simulink model "Output_ROS"  (R2022b)
settings: Solver=FixedStepAuto  StartTime=0.0  StopTime=128  FixedStep=0.02  RelTol=1e-3
undefined symbols (not defined in the file): b, unicycle, X, Y
libraries: robotlib x3, simulink_extras x1
settings Model: Creator=mustacchim  LastModifiedBy=mustacchim
settings OptimizationCC: EnhancedBackFolding=on  PassReuseOutputArgsAs=Individual arguments  ZeroExternalMemoryAtStartup=off  ZeroInternalMemoryAtStartup=off  MaxStackSize=64  OptimizeBlockOrder=speed  DifferentSizesBufferReuse=on  OptimizationCustomize=off  EfficientTunableParamExpr=on
settings DebuggingCC: ParameterTunabilityLossMsg=error
settings HardwareCC: ProdBitPerPointer=32  ProdBitPerSizeT=32  ProdBitPerPtrDiffT=32  ProdLargestAtomicFloat=None  ProdIntDivRoundTo=Undefined  ProdEndianess=Unspecified  ProdWordSize=32  ProdHWDeviceType=Generic->Unspecified (assume 32-bit Generic)
settings SFSimCC: MATLABDynamicMemAlloc=off
settings RTWCC: Description=Embedded Coder  SystemTargetFile=ert.tlc  HardwareBoard=Robot Operating System (ROS)  TLCOptions="-aInlineSetEventsForThisBaseRateFcn=TLC_FALSE -aSuppressMultiTaskScheduler=TLC_FALSE  -aRateBasedStepFcn=0"  TemplateMakefile=ert_default_tmf  Toolchain=Catkin  TargetLang=C++
settings CodeAppCC: ForceParamTrailComments=on  IgnoreCustomStorageClasses=off  OperatorAnnotations=on  SimulinkDataObjDesc=on  SFDataObjDesc=on  InsertBlockDesc=on

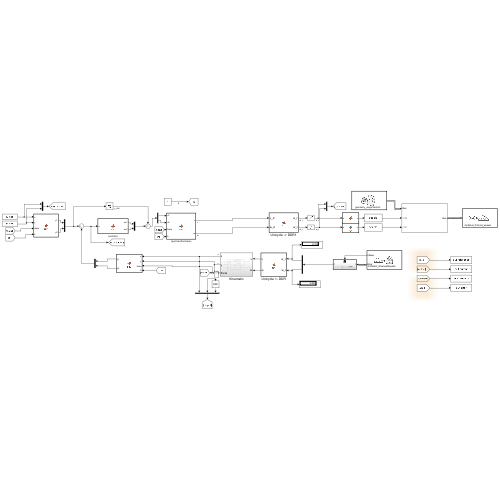
[thumbnail: Simulink's stored preview of the top-level diagram]
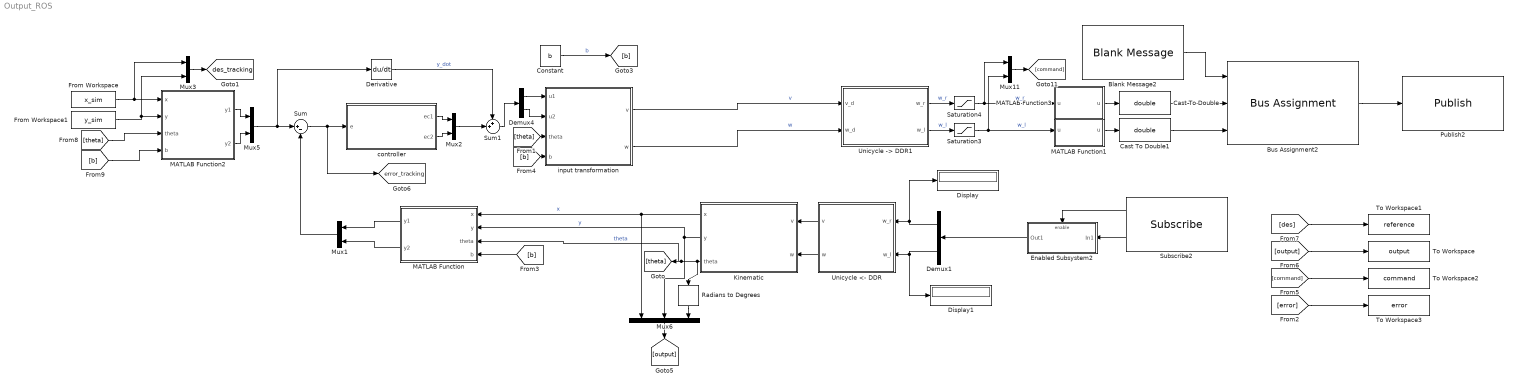
== system Output_ROS ==
  Blank Message2 : robotlib/Blank Message  messageClass=Message  entityType=geometry_msgs/Vector3  messageType=geometry_msgs/Vector3  SampleTime=0.02  legacyBusStruct=off
      settings: LibrarySourceBlock=roslib/ROS/Blank Message
  Bus Assignment2 : BusAssignment  AssignedSignals=X,Y
  Cast To Double : DataTypeConversion  OutDataTypeStr=double  SaturateOnIntegerOverflow=off  RndMeth=Floor
  Cast To Double1 : DataTypeConversion  OutDataTypeStr=double  SaturateOnIntegerOverflow=off  RndMeth=Floor
  Constant : Constant  Value=b
  Demux1 : Demux  Outputs=2
  Demux4 : Demux  Outputs=2
  Derivative : Derivative
  Display : Display
  Display1 : Display
  Enabled Subsystem2 : Subsystem  TreatAsAtomicUnit=on
  From Workspace : FromWorkspace  VariableName=x_sim
  From Workspace1 : FromWorkspace  VariableName=y_sim
  Kinematic : Subsystem
  MATLAB Function : MATLAB Function  TreatAsAtomicUnit=on
  MATLAB Function1 : MATLAB Function  TreatAsAtomicUnit=on
  MATLAB Function2 : MATLAB Function  TreatAsAtomicUnit=on
  MATLAB Function3 : MATLAB Function  TreatAsAtomicUnit=on
  Mux{1..3,5,11} (5 alike) : Mux  Inputs=2
  Mux6 : Mux  Inputs=3
  Publish2 : robotlib/Publish  topicSource=Select from ROS network  topic=/turtlebot_03/cmd_wheels  messageType=geometry_msgs/Vector3  legacyBusStruct=off  messageQueueLength=1
      settings: LibrarySourceBlock=roslib/ROS/Publish
  Radians to Degrees : simulink_extras/Transformations/Radians to Degrees
  Saturation3 : Saturate  UpperLimit=8  LowerLimit=-8
  Saturation4 : Saturate  UpperLimit=8  LowerLimit=-8
  Subscribe2 : robotlib/Subscribe  topicSource=Select from ROS network  topic=/turtlebot_03/wheelSpeeds  messageType=geometry_msgs/Vector3  SampleTime=0.02  legacyBusStruct=off  messageQueueLength=1
      settings: LibrarySourceBlock=roslib/ROS/Subscribe
  Sum : Sum  Inputs=|+-
  Sum1 : Sum  Inputs=++|
  To Workspace : ToWorkspace  VariableName=output  SaveFormat=Structure With Time  SampleTime=-1
  To Workspace1 : ToWorkspace  VariableName=reference  SaveFormat=Structure With Time  SampleTime=-1
  To Workspace2 : ToWorkspace  VariableName=command  SaveFormat=Structure With Time  SampleTime=-1
  To Workspace3 : ToWorkspace  VariableName=error  SaveFormat=Structure With Time  SampleTime=-1
  "Unicycle -> DDR1" : MATLAB Function  TreatAsAtomicUnit=on
  Unicycle <- DDR : MATLAB Function  TreatAsAtomicUnit=on
  controller : MATLAB Function  TreatAsAtomicUnit=on
  input transformation : MATLAB Function  TreatAsAtomicUnit=on
  tag scope: des_tracking=global, error_tracking=global
  wires:
  Demux4/2 -> input transformation/2(u2)
  [b] -> input transformation/4(b)
  Mux2/1 -> Sum1/2
  MATLAB Function2/2(y2) -> Mux5/2
  [b] -> MATLAB Function/4(b)
  [theta] -> input transformation/3(theta)
  MATLAB Function2/1(y1) -> Mux5/1
  From Workspace1/1 -> Mux3/2, MATLAB Function2/2(y)
  Mux3/1 -> [des_tracking]
  From Workspace/1 -> Mux3/1, MATLAB Function2/1(x)
  controller/1(ec1) -> Mux2/1
  input transformation/1(v) -> "Unicycle -> DDR1"/1(v_d)  "v"
  MATLAB Function/1(y1) -> Mux1/1
  controller/2(ec2) -> Mux2/2
  [b] -> MATLAB Function2/4(b)
  Sum1/1 -> Demux4/1
  Constant/1 -> [b]  "b"
  input transformation/2(w) -> "Unicycle -> DDR1"/2(w_d)  "w"
  Sum/1 -> [error_tracking], controller/1(e)
  MATLAB Function/2(y2) -> Mux1/2
  Derivative/1 -> Sum1/1  "y_dot"
  Mux1/1 -> Sum/2
  Demux4/1 -> input transformation/1(u1)
  [theta] -> MATLAB Function2/3(theta)
  Mux5/1 -> Derivative/1, Sum/1
  Cast To Double1/1 -> Bus Assignment2/3
  Cast To Double/1 -> Bus Assignment2/2
  Mux6/1 -> [output]
  Kinematic/1(x) -> MATLAB Function/1(x), Mux6/1  "x"
  Subscribe2/1 -> Enabled Subsystem2/Enable
  MATLAB Function3/1(u) -> Cast To Double/1
  Kinematic/3(theta) -> MATLAB Function/3(theta), [theta], Radians to Degrees/1  "theta"
  Mux11/1 -> [command]
  MATLAB Function1/1(u) -> Cast To Double1/1
  Radians to Degrees/1 -> Mux6/3
  Enabled Subsystem2/1(Out1) -> Demux1/1
  Bus Assignment2/1 -> Publish2/1
  Demux1/2 -> Display1/1, Unicycle <- DDR/2(w_l)
  Demux1/1 -> Display/1, Unicycle <- DDR/1(w_r)
  Saturation3/1 -> MATLAB Function1/1("u "), Mux11/2  "w_l"
  Saturation4/1 -> MATLAB Function3/1("u "), Mux11/1  "w_r"
  Unicycle <- DDR/2(w) -> Kinematic/2(w)
  Subscribe2/2 -> Enabled Subsystem2/1(In1)
  Unicycle <- DDR/1(v) -> Kinematic/1(v)
  "Unicycle -> DDR1"/1(w_r) -> Saturation4/1  "w_r"
  "Unicycle -> DDR1"/2(w_l) -> Saturation3/1  "w_l"
  [output] -> To Workspace/1
  Blank Message2/1 -> Bus Assignment2/1
  [des] -> To Workspace1/1
  [command] -> To Workspace2/1
  Kinematic/2(y) -> MATLAB Function/2(y), Mux6/2  "y"
  [error] -> To Workspace3/1

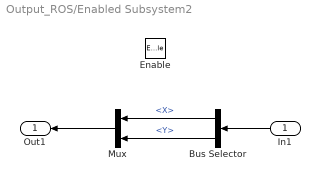
== system Output_ROS/Enabled Subsystem2 ==
  In1 : Inport
  Enable : EnablePort
  Bus Selector : BusSelector  OutputSignals=X,Y
  Mux : Mux  Inputs=2
  Out1 : Outport
  wires:
  Mux/1 -> Out1/1
  Bus Selector/1 -> Mux/1  "<X>"
  Bus Selector/2 -> Mux/2  "<Y>"
  In1/1 -> Bus Selector/1

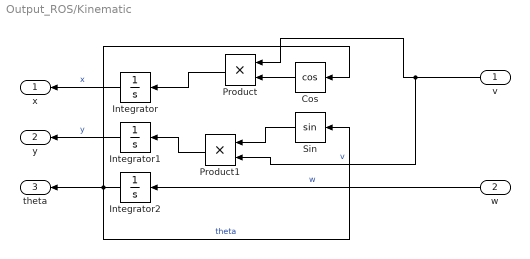
== system Output_ROS/Kinematic ==
  v : Inport
  w : Inport  Port=2
  Cos : Trigonometry  Operator=cos
  Integrator : Integrator  InitialCondition=unicycle.ic.x
  Integrator1 : Integrator  InitialCondition=unicycle.ic.y
  Integrator2 : Integrator  InitialCondition=unicycle.ic.theta
  Product : Product
  Product1 : Product
  Sin : Trigonometry
  x : Outport
  y : Outport  Port=2
  theta : Outport  Port=3
  wires:
  w/1 -> Integrator2/1  "w"
  Product/1 -> Integrator/1
  v/1 -> Product/1, Product1/2  "v"
  Cos/1 -> Product/2
  Integrator1/1 -> y/1  "y"
  Integrator/1 -> x/1  "x"
  Integrator2/1 -> theta/1, Sin/1, Cos/1  "theta"
  Product1/1 -> Integrator1/1
  Sin/1 -> Product1/1

== matlab function Output_ROS/MATLAB Function ==
  data: x input; y1 output; y input; theta input; b input; y2 output
function [y1,y2] = p2y(x,y,theta,b)

    y1 = x + b*cos(theta);
    y2 = y + b*sin(theta);
    
end

== matlab function Output_ROS/MATLAB Function1 ==
  data: u input; u output
function u = fcn(u)


    if (isnan(u))
        u = 0.1;
    end

end

== matlab function Output_ROS/MATLAB Function3 ==
  data: u input; u output
function u = fcn(u)

    if (isnan(u))
        u = 0.1;
    end

end

== matlab function Output_ROS/MATLAB Function2 ==
  data: x input; y1 output; y input; y2 output; theta input; b input
function [y1,y2] = p2y(x,y,theta,b)

y1 = x + b*cos(theta);
y2 = y + b*sin(theta);

== matlab function Output_ROS/controller ==
  data: e input; ec1 output; ec2 output
function [ec1, ec2] = fcn(e)

    %#codegen
    coder.extrinsic('evalin')
    k1 = 0;                  % Needed in order to set variable class correctly
    k2 = 0;                  % Needed in order to set variable class correctly
    k1 = evalin('base','k1'); % Read value from workspace
    k2 = evalin('base','k2'); % Read value from workspace
    
    ec1 = k1*(e(1));
    ec2 = k2*(e(2));
    
end

== matlab function Output_ROS/Unicycle <- DDR ==
  data: w_r input; v output; w_l input; w output
function [v, w] = fcn(w_r, w_l)

    %#codegen
    coder.extrinsic('evalin')
    d = 0;                  % Needed in order to set variable class correctly
    r = 0;                  % Needed in order to set variable class correctly
    d = evalin('base','unicycle.d'); % Read value from workspace
    r = evalin('base','unicycle.r'); % Read value from workspace

    v = r*(w_r + w_l)/2; % rad/s
    w = r*(w_r - w_l)/d; % rad/s

end

== matlab function Output_ROS/input transformation ==
  data: u1 input; u2 input; theta input; v output; b input; w output
function [v,w] = fcn(u1, u2, theta, b)

    R = [cos(theta),      sin(theta);
         -sin(theta)/b, cos(theta)/b];
    
    v = cos(theta)*u1 + sin(theta)*u2;
    w = (-sin(theta)/b)*u1 + (cos(theta)/b)*u2;

end

== matlab function Output_ROS/Unicycle -> DDR1 ==
  data: v_d input; w_r output; w_d input; w_l output
function [w_r, w_l] = fcn(v_d, w_d)

    %#codegen
    coder.extrinsic('evalin')
    d = 0;                  % Needed in order to set variable class correctly
    r = 0;                  % Needed in order to set variable class correctly
    d = evalin('base','unicycle.d'); % Read value from workspace
    r = evalin('base','unicycle.r'); % Read value from workspace

    w_r = ((2 * v_d) + (w_d * d)) / (2 * r);
    w_l = ((2 * v_d) - (w_d * d)) / (2 * r);

end
